simulink model "btns"  (R2018b)
settings: Solver=FixedStepDiscrete  StartTime=0.0  StopTime=10.0  FixedStep=0.1  RelTol=1e-3
settings Model: ExtModeTrigDuration=2  Creator=sin29  LastModifiedBy=sin29
settings SolverCC: AutoInsertRateTranBlk=on
settings DataIOCC: LimitDataPoints=on
settings OptimizationCC: DefaultParameterBehavior=Inlined  UseDivisionForNetSlopeComputation=on  UseFloatMulNetSlope=on  InlineInvariantSignals=on  PassReuseOutputArgsAs=Individual arguments  ZeroExternalMemoryAtStartup=off  ZeroInternalMemoryAtStartup=off  NoFixptDivByZeroProtection=on  EfficientFloat2IntCast=on  LifeSpan=1  MaxStackSize=64  OptimizeBlockOrder=speed  DifferentSizesBufferReuse=on
settings DebuggingCC: ParameterTunabilityLossMsg=error  AllowSymbolicDim=off  SFUnexpectedBacktrackingDiag=warning  SFNoUnconditionalDefaultTransitionDiag=warning  SFExecutionAtInitializationDiag=none
settings HardwareCC: ProdBitPerInt=16  ProdBitPerPointer=16  ProdBitPerSizeT=16  ProdBitPerPtrDiffT=16  ProdLargestAtomicFloat=None  ProdWordSize=8  ProdLongLongMode=on  ProdHWDeviceType=Atmel->AVR
settings SFSimCC: SimUseLocalCustomCode=off  MATLABDynamicMemAlloc=off
settings RTWCC: SystemTargetFile=ert.tlc  HardwareBoard=Arduino Uno  TemplateMakefile=ert_default_tmf  GenerateReport=on  RTWUseLocalCustomCode=off  Toolchain=Arduino AVR  BuildConfiguration=Faster Runs  IncludeHyperlinkInReport=on  LaunchReport=on  GenerateTraceInfo=on  GenerateTraceReport=on  GenerateTraceReportSl=on  GenerateTraceReportSf=on  GenerateTraceReportEml=on  GenerateCodeMetricsReport=on
settings CodeAppCC: ForceParamTrailComments=on  IgnoreCustomStorageClasses=off  OperatorAnnotations=on  SimulinkDataObjDesc=on  SFDataObjDesc=on  CustomSymbolStrGlobalVar=rt$N$M  CustomSymbolStrType=$N$M  CustomSymbolStrFcn=$N$M$F  CustomSymbolStrMacro=$N$M  InsertBlockDesc=on
settings ERTTargetCC: IncludeMdlTerminateFcn=off  CombineSignalStateStructs=on  SupportAbsoluteTime=off  SupportComplex=off  SupportNonInlinedSFcns=on  InlinedParameterPlacement=NonHierarchical  ERTFilePackagingFormat=CompactWithDataFile
settings ConfigComp: CovMetricSettings=dw  CovHtmlReporting=on  CovSaveCumulativeToWorkspaceVar=on  CovSaveSingleToWorkspaceVar=on  CovShowResultsExplorer=off  CovExternalEMLEnable=off  CovSFcnEnable=off

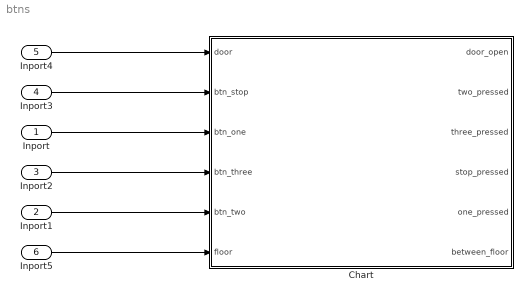
== system btns ==
  Inport : Inport
  Inport1 : Inport  Port=2
  Inport2 : Inport  Port=3
  Inport3 : Inport  Port=4
  Inport4 : Inport  Port=5
  Inport5 : Inport  Port=6
  Chart : Stateflow chart  TreatAsAtomicUnit=on
  wires:
  Inport/1 -> Chart/3(btn_one)
  Inport2/1 -> Chart/4(btn_three)
  Inport1/1 -> Chart/5(btn_two)
  Inport3/1 -> Chart/2(btn_stop)
  Inport4/1 -> Chart/1(door)
  Inport5/1 -> Chart/6(floor)

== stateflow chart btns/Chart ==
  state Reset
    entry:
    one_pressed = 0;
    two_pressed = 0;
    three_pressed = 0;
    door_open = 0;
    stop_pressed = 0;
  state two_bounce
  state three_bounce
  state stop_bounce
  state one_bounce
  state door_bounce
  state floor_bounce
  state floor_pos
    entry :
    between_floor = 1;
  state two_press
    entry:
    two_pressed = 1;
  state stop_press
    entry:
    stop_pressed =1 ;
  state three_press
    entry:
    three_pressed = 1;
  state door_status
    entry:
    door_open = 1;
  state one_press
    entry:
    one_pressed = 1;
  floor_pos -> Reset
  floor_bounce -> Reset [order 1] : [floor == 0]
  Reset -> floor_bounce [order 6] : [floor == 1]
  (default) -> Reset
  stop_press -> Reset
  one_press -> Reset
  Reset -> one_bounce [order 5] : [btn_one == 1]
  stop_bounce -> Reset [order 2] : [btn_stop == 0]
  one_bounce -> Reset [order 2] : [btn_one == 0]
  two_bounce -> Reset [order 2] : [btn_two == 0]
  Reset -> stop_bounce [order 4] : [btn_stop == 1]
  Reset -> two_bounce [order 1] : [btn_two == 1]
  door_bounce -> Reset [order 2] : [door == 0]
  two_press -> Reset
  three_bounce -> Reset [order 2] : [btn_three == 0]
  Reset -> three_bounce [order 2] : [btn_three== 1]
  three_press -> Reset
  door_status -> Reset
  Reset -> door_bounce [order 3] : [door == 1]
  two_bounce -> two_press [order 1] : [btn_two == 1&&after(0.2,msec)]
  three_bounce -> three_press [order 1] : [btn_three == 1&&after(0.2,msec)]
  stop_bounce -> stop_press [order 1] : [btn_stop == 1&&after(0.2,msec)]
  one_bounce -> one_press [order 1] : [btn_one == 1&&after(0.2,msec)]
  door_bounce -> door_status [order 1] : [door == 1&&after(0.2,msec)]
  floor_bounce -> floor_pos [order 2] : [floor == 1&&after(0.2,msec)]
  data: door input; btn_stop input; btn_one input; btn_three input; btn_two input; door_open output; two_pressed output; three_pressed output; stop_pressed output; one_pressed output; between_floor output; floor input
